simulink model "Satellite_Attitude_Control_Scenario_B"  (R2026a)
settings: Solver=VariableStepAuto  StopTime=25
libraries: slpidlib x1
settings Model: Creator=sreecharan  LastModifiedBy=sreecharan

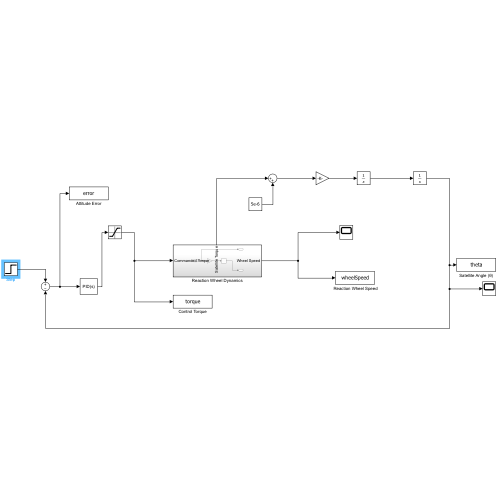
[thumbnail: Simulink's stored preview of the top-level diagram]
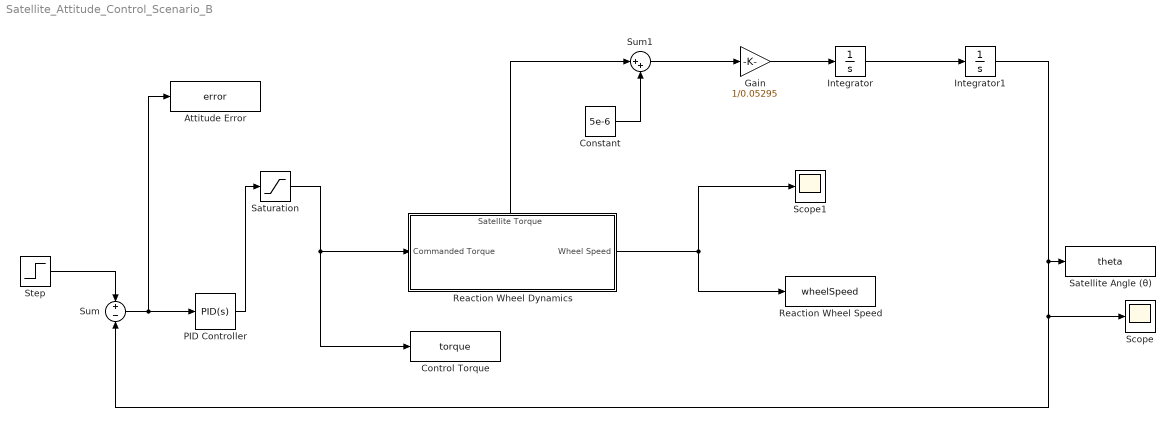
== system Satellite_Attitude_Control_Scenario_B ==
  " Reaction Wheel Speed" : ToWorkspace  VariableName=wheelSpeed  SampleTime=-1
  Attitude Error : ToWorkspace  VariableName=error  SampleTime=-1
  Constant : Constant  Value=5e-6
  Control Torque : ToWorkspace  VariableName=torque  SampleTime=-1
  Gain : Gain  Gain=1/0.05295
  Integrator : Integrator
  Integrator1 : Integrator
  PID Controller : slpidlib/PID Controller  Controller=PID  Form=Parallel  TimeDomain=Continuous-time  UseExternalTs=off  SampleTime=-1  IntegratorMethod=Forward Euler  FilterMethod=Forward Euler  ControllerParametersSource=internal  P=0.08  I=0.009  UseKiTs=off  D=0.17  UseExternalDerivativeSource=off  N=100  UseFilter=on  TunerSelectOption=Transfer Function Based (PID Tuner App)  InitialConditionSource=internal  InitialConditionForIntegrator=0  InitialConditionForFilter=0  DifferentiatorICPrevScaledInput=0  ExternalReset=none  TrackingMode=off  Kt=1  LimitOutput=off  SatLimitsSource=internal  UpperSaturationLimit=inf  LowerSaturationLimit=-inf  LinearizeAsGain=on  AntiWindupMode=none  Kb=1  LimitIntegrator=off  UpperIntegratorSaturationLimit=inf  LowerIntegratorSaturationLimit=-inf  POutMin=[]  POutMax=[]  IOutMin=[]  IOutMax=[]  DOutMin=[]  DOutMax=[]  NOutMin=[]  NOutMax=[]  SumOutMin=[]  SumOutMax=[]  SaturationOutMin=[]  SaturationOutMax=[]  PParamMin=[]  PParamMax=[]  IParamMin=[]  IParamMax=[]  DParamMin=[]  DParamMax=[]  NParamMin=[]  NParamMax=[]  KbParamMin=[]  KbParamMax=[]  KtParamMin=[]  KtParamMax=[]  KbOutMin=[]  KbOutMax=[]  KtOutMin=[]  KtOutMax=[]  IntegratorOutMin=[]  IntegratorOutMax=[]  FilterOutMin=[]  FilterOutMax=[]  SumI1OutMin=[]  SumI1OutMax=[]  SumI2OutMin=[]  SumI2OutMax=[]  SumI3OutMin=[]  SumI3OutMax=[]  SumI4OutMin=[]  SumI4OutMax=[]  SumDOutMin=[]  SumDOutMax=[]  DifferentiatorOutMin=[]  DifferentiatorOutMax=[]  FilterDiffOutCoefMin=[]  FilterDiffOutCoefMax=[]  ReciprocalOutMin=[]  ReciprocalOutMax=[]  SumDenOutMin=[]  SumDenOutMax=[]  SumNumOutMin=[]  SumNumOutMax=[]  DivideOutMin=[]  DivideOutMax=[]  UdiffTsProdOutMin=[]  UdiffTsProdOutMax=[]  NTsProdOutMin=[]  NTsProdOutMax=[]  UintegralTsProdOutMin=[]  UintegralTsProdOutMax=[]  UngainTsProdOutMin=[]  UngainTsProdOutMax=[]  ClampingZeroOutDataTypeStr=Inherit: Inherit via back propagation  ClampingZeroOutMin=[]  ClampingZeroOutMax=[]  FilterDenConstantOutDataTypeStr=Inherit: Inherit via back propagation  FilterDenConstantOutMin=[]  FilterDenConstantOutMax=[]  PCopyOutDataTypeStr=Inherit: Inherit via back propagation  PCopyOutMin=[]  PCopyOutMax=[]  NCopyOutDataTypeStr=Inherit: Inherit via back propagation  NCopyOutMin=[]  NCopyOutMax=[]  IntegratorContinuousStateAttributes=''  IntegratorStateMustResolveToSignalObject=off  IntegratorRTWStateStorageClass=Auto  FilterContinuousStateAttributes=''  FilterStateMustResolveToSignalObject=off  FilterRTWStateStorageClass=Auto  ParallelPVariant=InternalParameters  IdealPVariant=Disabled  IVariant=InternalParameters  DVariant=InternalParameters  IntegratorVariant=Continuous  SatVariant=Disabled  AWVariant=Passthrough  PCopyVariant=Disabled  TRVariant=Disabled  FdbkBlocksVariant=Forward  IdealPFdbkVariant=Disabled  SatFdbkVariant=Disabled  DerivativeFilterVariant=ContFilter  NVariant=InternalParameters  NCopyVariant=Disabled  FilterICVariant=InternalICsFilter  IntegratorICVariant=InternalICs  ExternalResetVariant=Disabled  TRSumVariant=Passthrough  SumFdbkVariant=Disabled  SumVariant=Sum_PID  TsampFilterVariant=InternalTs  TsampNgainVariant=Passthrough  TsampIntegralVariant=Disabled_SignalSpec  ExternalSaturationOutDataTypeStr=Inherit: Same as second input  DerivativeSourceVariant=ErrorSignal  PreIntVariant=InternalPreInt
  Reaction Wheel Dynamics : Subsystem
      settings: PortSchema="{\"entries\":[{\"content\":{\"sides\":[{\"content\":{\"connectorIds\":[\"In1\"]},\"type\":\"ConnectorPlacement.EquallySpacedRectSide\",\"uuid\":\"5dbcf71b-4bbb-463b-beea-80ab16e1a559\"},{\"content\":{\"connectorIds\":[\"Out1\"],\"side\":\"RIGHT\"},\"type\":\"ConnectorPlacement.EquallySpacedRectSide\",\"uuid\":\"2ea40819-5353-4131-8956-55917f52d00c\"},{\"content\":{\"connectorIds\":[\"Out2\"],\"side\":\"TOP\"},\"type\":\"ConnectorPlacement.EquallySpacedRectSide\",\"uuid\":\"c59e7123-e0d0-45cb-aaed-c6c85372aea0\"}]},\"type\":\"ConnectorPlacement.EquallySpacedConnector\",\"uuid\":\"1d5021f4-2059-4a45-8503-4e7cffae7b0a\"}],\"packageUris\":[\"http://schema.mathworks.com/mf0/Connector/R2020b\"],\"version\":\"1.0\"}"
  Satellite Angle (θ) : ToWorkspace  VariableName=theta  SampleTime=-1
  Saturation : Saturate  UpperLimit=0.03  LowerLimit=-0.03
  Scope : Scope
      settings: ActiveDisplayYMinimum=-117.08314608632352  ActiveDisplayYMaximum=139.43639900394709
  Scope1 : Scope
      settings: ActiveDisplayYMinimum=-1  ActiveDisplayYMaximum=1
  Step : Step  FinalValue=pi/4  SampleTime=0
  Sum : Sum  Inputs=+-
  Sum1 : Sum  Inputs=|++
  wires:
  Step/1 -> Sum/1
  Sum/1 -> PID Controller/1, Attitude Error/1
  Gain/1 -> Integrator/1
  Integrator/1 -> Integrator1/1
  Integrator1/1 -> Scope/1, Sum/2, Satellite Angle (θ)/1
  PID Controller/1 -> Saturation/1
  Reaction Wheel Dynamics/1(Wheel Speed) -> Scope1/1, " Reaction Wheel Speed"/1
  Saturation/1 -> Control Torque/1, Reaction Wheel Dynamics/1(Commanded Torque)
  Reaction Wheel Dynamics/2(Satellite Torque) -> Sum1/1
  Constant/1 -> Sum1/2
  Sum1/1 -> Gain/1

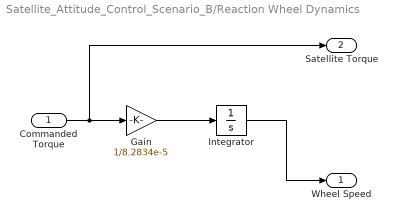
== system Satellite_Attitude_Control_Scenario_B/Reaction Wheel Dynamics ==
  Commanded Torque : Inport
  Gain : Gain  Gain=1/8.2834e-5
  Integrator : Integrator
  Wheel Speed : Outport
  Satellite Torque : Outport  Port=2
  wires:
  Commanded Torque/1 -> Satellite Torque/1, Gain/1
  Gain/1 -> Integrator/1
  Integrator/1 -> Wheel Speed/1
